simulink model "Daolibai_design_OSFandPIOFtu"  (R2016a)
settings: Solver=VariableStepAuto  SolverMode=SingleTasking  StartTime=0.0  StopTime=50  RelTol=1e-3
values from neighbouring files (symbols this model uses):
  A = [-18/7 9 0;1 -1 1;0 -14.28 0]    [Caishidianlu_design.m]    (also in Daolibai_analysis_ControllAndObserv.m = [0 1 0 0; Daolibai_analysis_stability.m = [0 1 0 0; Daolibai_design_OSF.m = [0 1 0 0; Daolibai_design_OSFandPIOF.m = [0 1 0 0)
  B = [27/7;0;0]    [Caishidianlu_design.m]    (also in Daolibai_analysis_ControllAndObserv.m = [0;1;0;-2]; Daolibai_analysis_stability.m = [0;1;0;-2]; Daolibai_design_OSF.m = [0;1;0;-2]; Daolibai_design_OSFandPIOF.m = [0;1;0;-2])
  C = [1 0 0]    [Caishidianlu_design.m]    (also in Daolibai_analysis_ControllAndObserv.m = [1 0 0 0]; Daolibai_analysis_stability.m = [1 0 0 0]; Daolibai_design_OSF.m = [1 0 0 0]; Daolibai_design_OSFandPIOF.m = [1 0 0 0])
  D = [1 0 0]    [Caishidianlu_design.m]    (also in Daolibai_analysis_ControllAndObserv.m = [0]; Daolibai_analysis_stability.m = [0]; Daolibai_design_OSF.m = [0]; Daolibai_design_OSFandPIOF.m = [0])
  G = G'    [Daolibai_design_OSF.m]    (also in Daolibai_design_OSFandPIOF.m)
  Init = [0.1 0.1 0.5 0.5]    [Daolibai_design_OSF.m]    (also in Daolibai_design_OSFandPIOF.m = [0 0.04 0.005 0.1 ]; Daolibai_design_SFandOF.m; Daolibai_design_SFandPIOF.m = [0 0.1 0.005 0.1 ])
  Initobserv = [0.1 0.1 0.4 0.3]    [Daolibai_design_OSF.m]    (also in Daolibai_design_OSFandPIOF.m = [0 0.015 0 0.1])
  K1 = K(:,1:4)    [Daolibai_design_OSFandPIOF.m]    (also in Daolibai_design_SFandPIOF.m)
  K2 = -K(:,5:5)    [Daolibai_design_OSFandPIOF.m]    (also in Daolibai_design_SFandPIOF.m)
settings Model: Creator=19017  LastModifiedBy=19017
settings DataIOCC: ReturnWorkspaceOutputs=on
settings DebuggingCC: SFUnexpectedBacktrackingDiag=error  SFNoUnconditionalDefaultTransitionDiag=error
settings SFSimCC: SimUseLocalCustomCode=on
settings RTWCC: RTWUseLocalCustomCode=on
settings GRTTargetCC: TargetLangStandard=C99 (ISO)
settings ConfigComp: CovMetricSettings=dwe  CovSaveCumulativeToWorkspaceVar=off  CovSaveSingleToWorkspaceVar=off  CovExternalEMLEnable=on

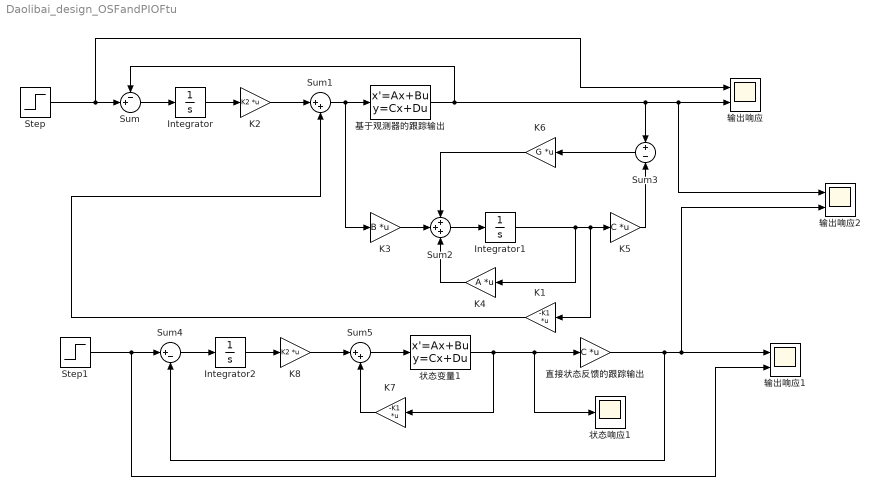
== system Daolibai_design_OSFandPIOFtu ==
  Integrator : Integrator  InitialCondition=[0]
  Integrator1 : Integrator  InitialCondition=Initobserv
  Integrator2 : Integrator  InitialCondition=[0]
  K1 : Gain  Gain=-K1  Multiplication=Matrix(K*u)
  K2 : Gain  Gain=K2  Multiplication=Matrix(K*u)
  K3 : Gain  Gain=B  Multiplication=Matrix(K*u)
  K4 : Gain  Gain=A  Multiplication=Matrix(K*u)
  K5 : Gain  Gain=C  Multiplication=Matrix(K*u)
  K6 : Gain  Gain=G  Multiplication=Matrix(K*u)
  K7 : Gain  Gain=-K1  Multiplication=Matrix(K*u)
  K8 : Gain  Gain=K2  Multiplication=Matrix(K*u)
  Step : Step  SampleTime=0
  Step1 : Step  SampleTime=0
  Sum : Sum  Inputs=-+|
  Sum1 : Sum  Inputs=|++
  Sum2 : Sum  Inputs=+++
  Sum3 : Sum  Inputs=+|-
  Sum4 : Sum  Inputs=|+-
  Sum5 : Sum  Inputs=|++
  基于观测器的跟踪输出 : StateSpace  A=A  B=B  C=C  D=D  X0=Init
  状态变量1 : StateSpace  A=A  B=B  C=eye(4)  D=[0;0;0;0]  X0=Init
  状态响应1 : Scope
  直接状态反馈的跟踪输出 : Gain  Gain=C  Multiplication=Matrix(K*u)
  输出响应 : Scope  NumInputPorts=2
  输出响应1 : Scope  NumInputPorts=2
  输出响应2 : Scope  NumInputPorts=2
  wires:
  基于观测器的跟踪输出/1 -> Sum3/1, 输出响应2/1, 输出响应/2, Sum/1
  Sum/1 -> Integrator/1
  Sum1/1 -> K3/1, 基于观测器的跟踪输出/1
  Step/1 -> 输出响应/1, Sum/2
  Integrator/1 -> K2/1
  Integrator1/1 -> K4/1, K1/1, K5/1
  K4/1 -> Sum2/3
  Sum2/1 -> Integrator1/1
  K3/1 -> Sum2/2
  K2/1 -> Sum1/1
  K1/1 -> Sum1/2
  K5/1 -> Sum3/2
  Sum3/1 -> K6/1
  K6/1 -> Sum2/1
  直接状态反馈的跟踪输出/1 -> Sum4/2, 输出响应2/2, 输出响应1/1
  Sum4/1 -> Integrator2/1
  K7/1 -> Sum5/2
  Sum5/1 -> 状态变量1/1
  Step1/1 -> 输出响应1/2, Sum4/1
  K8/1 -> Sum5/1
  Integrator2/1 -> K8/1
  状态变量1/1 -> 直接状态反馈的跟踪输出/1, 状态响应1/1, K7/1
